simulink model "DDC"  (R2025a)
settings: Solver=FixedStepAuto  StartTime=0.0  StopTime=inf  FixedStep=1/Fs  RelTol=1e-3
undefined symbols (not defined in the file): Fs, h
libraries: dspsrcs4 x1, dsphdlsigops2 x1
settings Model: Creator=gxoro  LastModifiedBy=gxoro

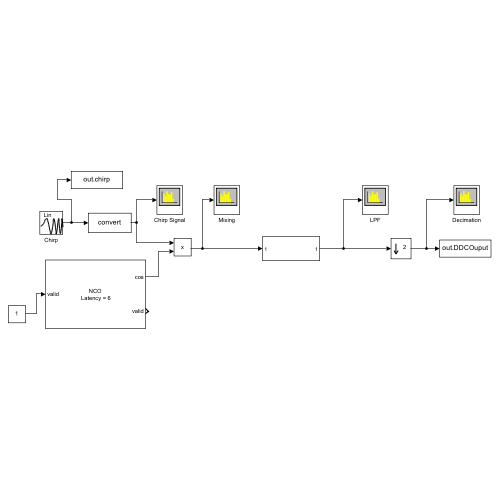
[thumbnail: Simulink's stored preview of the top-level diagram]
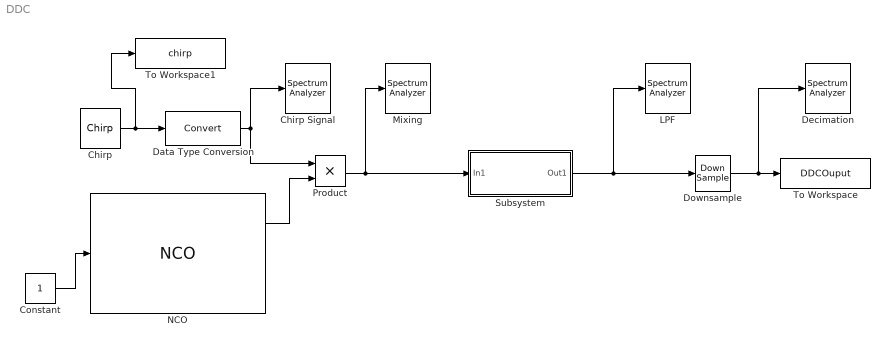
== system DDC ==
  Chirp : dspsrcs4/Chirp  sweep=Linear  mode=Unidirectional  f0=10e6  f1=20e6  t1=0.00001998  Tsweep=0.00001998  phase=0  Ts=1/1/Fs  spf=1  datatype=double  OutputFrames=off
  Chirp Signal : SpectrumAnalyzer  WindowPosition=[2.000000,458.000000,766.000000,377.000000,]  Visible=on  ScopeFrameLocation=window  WindowInvariantSamplesPerUpdate=on  Span=60000000  StartFrequency=-30000000  StopFrequency=30000000  YLimits=[-41.4607 7.3068]
  Constant : Constant  OutDataTypeStr=boolean  SampleTime=1/Fs
  Data Type Conversion : DataTypeConversion  SaturateOnIntegerOverflow=off  RndMeth=Floor
  Decimation : SpectrumAnalyzer  WindowPosition=[770.000000,50.000000,766.000000,377.000000,]  Visible=on  ScopeFrameLocation=window  WindowInvariantSamplesPerUpdate=on  Span=60000000  StartFrequency=-30000000  StopFrequency=30000000  YLimits=[-88.0062 5.9771]
  Downsample : DownSample  AllowArbitraryFixedInput=on
  LPF : SpectrumAnalyzer  WindowPosition=[2.000000,50.000000,766.000000,377.000000,]  Visible=on  ScopeFrameLocation=window  WindowInvariantSamplesPerUpdate=on  Span=60000000  StartFrequency=-30000000  StopFrequency=30000000  YLimits=[-141.7912 13.5098]
  Mixing : SpectrumAnalyzer  WindowPosition=[770.000000,458.000000,766.000000,377.000000,]  Visible=on  ScopeFrameLocation=window  WindowInvariantSamplesPerUpdate=on  Span=60000000  StartFrequency=-30000000  StopFrequency=30000000  YLimits=[-18.8566 1.3442]  SelectedToolstripTab=spectrumAnalyzerToolstrip.spectrumTab
  NCO : dsphdlsigops2/NCO  PhaseIncrementSource=Property  PhaseIncrement=phIncr  PhaseOffsetSource=Property  PhaseOffset=phOff  DitherSource=Property  NumDitherBits=dithBits  SamplesPerFrame=1  LUTCompress=off  ResetAction=off  Waveform=Cosine  PhasePort=off  SimulateUsing=Code generation  AccumulatorWL=N  PhaseQuantization=on  NumQuantizerAccumulatorBits=Q  OutputDataType=Binary point scaling  OutputWL=16  OutputFL=14
  Product : Product
  Subsystem : Subsystem
  To Workspace : ToWorkspace  VariableName=DDCOuput  SaveFormat=Timeseries  SampleTime=-1
  To Workspace1 : ToWorkspace  VariableName=chirp  SaveFormat=Timeseries  SampleTime=-1
  wires:
  NCO/1 -> Product/2
  Product/1 -> Subsystem/1(In1), Mixing/1
  Constant/1 -> NCO/1
  Subsystem/1(Out1) -> Downsample/1, LPF/1
  Downsample/1 -> Decimation/1, To Workspace/1
  Chirp/1 -> To Workspace1/1, Data Type Conversion/1
  Data Type Conversion/1 -> Chirp Signal/1, Product/1

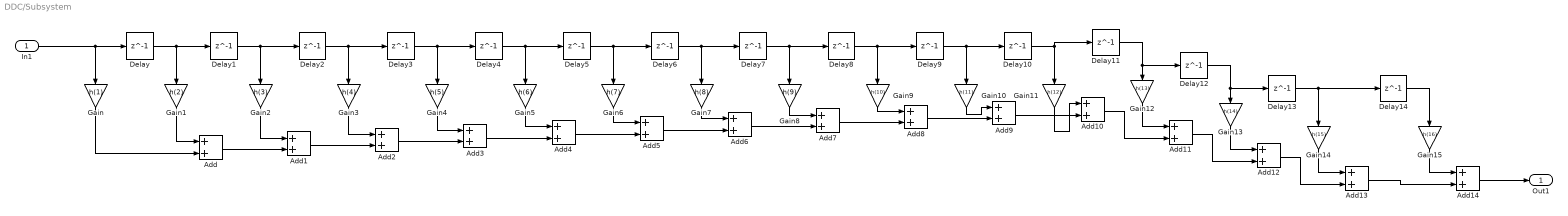
== system DDC/Subsystem ==
  In1 : Inport
  Add{,1..14} (15 alike) : Sum
  Delay{,1..14} (15 alike) : Delay  DelayLength=1  InitialCondition=0
  Gain : Gain  Gain=h(1)
  Gain1 : Gain  Gain=h(2)
  Gain10 : Gain  Gain=h(11)
  Gain11 : Gain  Gain=h(12)
  Gain12 : Gain  Gain=h(13)
  Gain13 : Gain  Gain=h(14)
  Gain14 : Gain  Gain=h(15)
  Gain15 : Gain  Gain=h(16)
  Gain2 : Gain  Gain=h(3)
  Gain3 : Gain  Gain=h(4)
  Gain4 : Gain  Gain=h(5)
  Gain5 : Gain  Gain=h(6)
  Gain6 : Gain  Gain=h(7)
  Gain7 : Gain  Gain=h(8)
  Gain8 : Gain  Gain=h(9)
  Gain9 : Gain  Gain=h(10)
  Out1 : Outport
  wires:
  In1/1 -> Delay/1, Gain/1
  Gain/1 -> Add/2
  Gain1/1 -> Add/1
  Delay/1 -> Delay1/1, Gain1/1
  Delay1/1 -> Gain2/1, Delay2/1
  Gain2/1 -> Add1/1
  Add/1 -> Add1/2
  Add1/1 -> Add2/2
  Gain3/1 -> Add2/1
  Delay2/1 -> Delay3/1, Gain3/1
  Add2/1 -> Add3/2
  Delay3/1 -> Delay4/1, Gain4/1
  Gain4/1 -> Add3/1
  Delay4/1 -> Delay5/1, Gain5/1
  Gain5/1 -> Add4/1
  Add3/1 -> Add4/2
  Delay5/1 -> Delay6/1, Gain6/1
  Gain6/1 -> Add5/1
  Add4/1 -> Add5/2
  Add5/1 -> Add6/2
  Delay6/1 -> Gain7/1, Delay7/1
  Gain7/1 -> Add6/1
  Add6/1 -> Add7/2
  Gain8/1 -> Add7/1
  Delay7/1 -> Delay8/1, Gain8/1
  Delay8/1 -> Delay9/1, Gain9/1
  Add7/1 -> Add8/2
  Gain9/1 -> Add8/1
  Gain10/1 -> Add9/1
  Delay9/1 -> Delay10/1, Gain10/1
  Add8/1 -> Add9/2
  Add9/1 -> Add10/2
  Delay10/1 -> Gain11/1, Delay11/1
  Gain11/1 -> Add10/1
  Gain12/1 -> Add11/1
  Add10/1 -> Add11/2
  Delay11/1 -> Delay12/1, Gain12/1
  Delay12/1 -> Delay13/1, Gain13/1
  Gain13/1 -> Add12/1
  Add11/1 -> Add12/2
  Delay13/1 -> Delay14/1, Gain14/1
  Add12/1 -> Add13/2
  Gain14/1 -> Add13/1
  Delay14/1 -> Gain15/1
  Add13/1 -> Add14/2
  Gain15/1 -> Add14/1
  Add14/1 -> Out1/1
